simulink model "basic"  (Simulink 7.7)
settings: Solver=ode45  StartTime=0.0  StopTime=10.0  RelTol=1e-3
settings Model: Creator=spu  LastModifiedBy=mestan

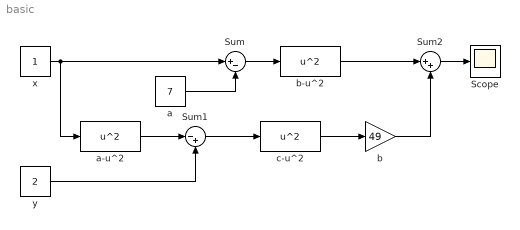
== system basic ==
  Scope : Scope
  Sum : Sum  Inputs=|+-
  Sum1 : Sum  Inputs=|-+
  Sum2 : Sum  Inputs=|++
  a : Constant  Value=7
  "a-u^2 " : MATLABFcn  MATLABFcn=u^2
  b : Gain  Gain=49
  b-u^2 : MATLABFcn  MATLABFcn=u^2
  c-u^2 : MATLABFcn  MATLABFcn=u^2
  x : Constant
  y : Constant  Value=2
  wires:
  Sum/1 -> b-u^2/1
  x/1 -> Sum/1, "a-u^2 "/1
  a/1 -> Sum/2
  y/1 -> Sum1/2
  Sum1/1 -> c-u^2/1
  c-u^2/1 -> b/1
  b-u^2/1 -> Sum2/1
  b/1 -> Sum2/2
  "a-u^2 "/1 -> Sum1/1
  Sum2/1 -> Scope/1
